simulink model "Openloop_mod"  (R2021a)
settings: Solver=VariableStepAuto  StartTime=0.0  StopTime=1  RelTol=1e-3
model workspace (MAT data in the model file):
  Vdc = 30
libraries: spsControlledVoltageSourceLib x1, spsGroundLib x1, spsPermanentMagnetSynchronousMachineLib x1, spsSawtoothGeneratorLib x1, spsThreePhaseVIMeasurementLib x1, spsUniversalBridgeLib x1, spsTriangleGeneratorLib x1, spspowerguiLib x1
settings Model: Creator=Zzx  LastModifiedBy=Zzx

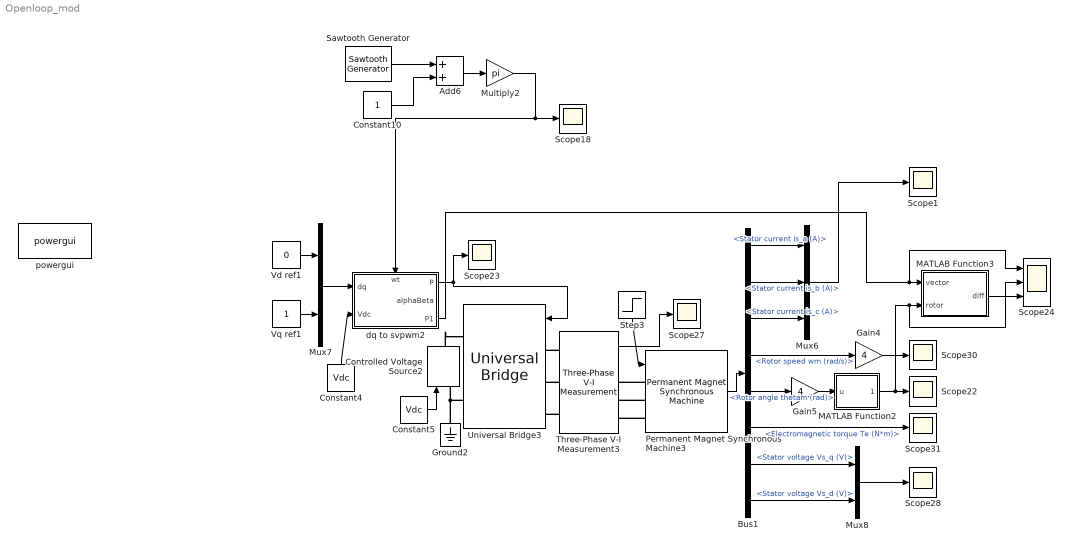
== system Openloop_mod ==
  Add6 : Sum
  Bus1 : BusSelector  OutputSignals=Stator current is_a (A),Stator current is_b (A),Stator current is_c (A),Rotor speed wm (rad/s),Rotor angle thetam (rad),Electromagnetic torque Te (N*m),Stator voltage Vs_q (V),Stator voltage Vs_d (V)
  Constant10 : Constant
  Constant4 : Constant  Value=Vdc
  Constant5 : Constant  Value=Vdc
  Controlled Voltage Source2 : spsControlledVoltageSourceLib/Controlled Voltage Source  Initialize=on  Source_Type=DC  Amplitude=0  Phase=0  Frequency=0  Measurements=Voltage
  Gain4 : Gain  Gain=4
  Gain5 : Gain  Gain=4
  Ground2 : spsGroundLib/Ground  LConnTagsString=a
  MATLAB Function2 : MATLAB Function  TreatAsAtomicUnit=on
  MATLAB Function3 : MATLAB Function  TreatAsAtomicUnit=on
  Multiply2 : Gain  Gain=pi
  Mux6 : Mux  Inputs=3
  Mux7 : Mux  Inputs=2
  Mux8 : Mux  Inputs=2
  Permanent Magnet Synchronous Machine3 : spsPermanentMagnetSynchronousMachineLib/Permanent Magnet Synchronous Machine  NbPhases=3  FluxDistribution=Sinusoidal  RotorType=Round  MechanicalLoad=Torque Tm  PresetModel=No  ShowDetailedParameters=on  MeasurementBus=off  Resistance=0.89  Inductance=8.5e-3  dqInductances=[8.5e-3,8.5e-3]  La=0.00062  MachineConstant=Voltage Constant (V_peak L-L / krpm)  Flux=0.0056925  VoltageCst=4.13  TorqueCst=0.034155  Flat=120  Mechanical=[ 0.8e-3, 0 4]  PolePairs=4  InitialConditions=[0,0, 0,0]  InitialConditions5ph=[0 0 0 0 0 0]  RefAngle=Aligned with phase A axis (original Park)  IterativeDiscreteModel=Trapezoidal non iterative  TsBlock=-1  TsPowergui=0
  Sawtooth Generator : spsSawtoothGeneratorLib/Sawtooth Generator  Freq=1  Phase=0  Ts=0
  Scope{1,18,22..23,27..28,30..31} (8 alike) : Scope
  Scope24 : Scope  NumInputPorts=3
  Step3 : Step  Time=0.5  After=0  SampleTime=0
  Three-Phase V-I Measurement3 : spsThreePhaseVIMeasurementLib/Three-Phase V-I Measurement  VoltageMeasurement=phase-to-ground  SetLabelV=off  LabelV=Vabc  Vpu=off  VpuLL=off  CurrentMeasurement=yes  SetLabelI=off  LabelI=Iabc  Ipu=off  Pbase=100e6  Vbase=500e3  OutputType=Complex  PhasorSimulation=off  PSBequivalent=0
  Universal Bridge3 : spsUniversalBridgeLib/Universal Bridge  Arms=3  SnubberResistance=1e5  SnubberCapacitance=inf  Device=IGBT / Diodes  Ron=1e-3  Lon=0  ForwardVoltages="[  0  0  ]"  ForwardVoltage=0  GTOparameters=[ 10e-6 , 20e-6 ]  IGBTparameters=[ 1e-6 , 2e-6 ]  Measurements=None  Measurements_2=None  converterType=Rectifier
  Vd ref1 : Constant  Value=0
  Vq ref1 : Constant
  dq to svpwm2 : Subsystem
      settings: PortSchema="{\"entries\":[{\"content\":{\"sides\":[{\"content\":{\"connectorIds\":[\"In1\",\"In2\"]},\"type\":\"ConnectorPlacement.EquallySpacedRectSide\",\"uuid\":\"e1c1c047-3402-4677-a9d9-6a01dbf7db4f\"},{\"content\":{\"connectorIds\":[\"Out1\",\"Out2\",\"Out3\"],\"side\":\"RIGHT\"},\"type\":\"ConnectorPlacement.EquallySpacedRectSide\",\"uuid\":\"6de788b8-e34e-4cfb-aebc-1ea17bcaea49\"},{\"content\":{\"connectorIds\":[\"In3\"],\"side\":\"TOP\"},\"type\":\"ConnectorPlacement.EquallySpacedRectSide\",\"uuid\":\"54a12e6c-3903-4ffc-a6c4-92faade7b32a\"},{\"content\":{\"connectorIds\":[],\"side\":\"BOTTOM\"},\"type\":\"ConnectorPlacement.EquallySpacedRectSide\",\"uuid\":\"2c718e0e-a6ab-4bdd-bca3-831c52d4e29e\"}]},\"type\":\"ConnectorPlacement.EquallySpacedConnector\",\"uuid\":\"b871e660-d5e9-497f-a8ea-54e97e14f77f\"}],\"packageUris\":[\"http://schema.mathworks.com/mf0/Connector/R2020b\"],\"version\":\"1.0\"}"
  powergui : spspowerguiLib/powergui  Priority=1  SimulationMode=Continuous  SampleTime=50e-6  frequency=60  Iterations=50  frequencyindice=0  Pbase=100e6  ErrMax=1e-4  UnitsV=kV  UnitsW=MW  buscounter=0  FunctionMessages=off  echomessages=off  EnableUseOfTLC=off  CurrentSourceSwitches=off  DisableSnubberDevices=off  DisableRonSwitches=off  DisableVfSwitches=off  DisplayEquations=off  AutomaticDiscreteSolvers=off  SolverType=Tustin/Backward Euler (TBE)  Interpol=off  ExternalGateDelay=off  methode=off  Ts=100  x0status=blocks  SPID=on  SwTol=0  HookPort=off  NonlinearTolerance=1e-4  nMaxIteration=100  ContinueOnMaxIteration=off  RestoreLinks=warning  ResistiveCurrentMeasurement=off  Frange=[0:2:500]  Ylog=off  Xlog=on  ShowGrid=off  save=off  variable=ZData  structure=0  ZoomFFT=off  StartTime=0.0  cycles=1  DisplayStyle=1  fundamental=60  FreqAxis=off  MaxFrequency=1000  frequencyindicesteady=1  RmsSteady=1  display=off
  wires:
  MATLAB Function3/1(diff) -> Scope24/3
  dq to svpwm2/3(P1) -> Scope24/1, MATLAB Function3/1(vector)
  Permanent Magnet Synchronous Machine3/1 -> Bus1/1
  dq to svpwm2/1(P) -> Universal Bridge3/1, Scope23/1
  MATLAB Function2/1(theta) -> Scope24/2, MATLAB Function3/2(rotor), Scope22/1
  Constant5/1 -> Controlled Voltage Source2/1
  Mux8/1 -> Scope28/1
  Bus1/1 -> Mux6/1  "<Stator current is_a (A)>"
  Vd ref1/1 -> Mux7/1
  Bus1/3 -> Mux6/3  "<Stator current is_c (A)>"
  Bus1/4 -> Gain4/1  "<Rotor speed wm (rad/s)>"
  Bus1/8 -> Mux8/2  "<Stator voltage Vs_d (V)>"
  Vq ref1/1 -> Mux7/2
  Mux7/1 -> dq to svpwm2/1(dq)
  Gain5/1 -> MATLAB Function2/1(u)
  Step3/1 -> Permanent Magnet Synchronous Machine3/1
  Bus1/5 -> Gain5/1  "<Rotor angle thetam (rad)>"
  Bus1/2 -> Mux6/2  "<Stator current is_b (A)>"
  Three-Phase V-I Measurement3/1 -> Scope27/1
  Sawtooth Generator/1 -> Add6/1
  Gain4/1 -> Scope30/1
  Add6/1 -> Multiply2/1
  Constant4/1 -> dq to svpwm2/2(Vdc)
  Multiply2/1 -> dq to svpwm2/3(wt), Scope18/1
  Constant10/1 -> Add6/2
  Bus1/6 -> Scope31/1  "<Electromagnetic torque Te (N*m)>"
  Bus1/7 -> Mux8/1  "<Stator voltage Vs_q (V)>"
  Mux6/1 -> Scope1/1
  connections:
  Universal Bridge3/RConn2 -- Controlled Voltage Source2/LConn1 -- Ground2/LConn1
  Permanent Magnet Synchronous Machine3/LConn2 -- Three-Phase V-I Measurement3/RConn2
  Three-Phase V-I Measurement3/LConn3 -- Universal Bridge3/LConn3
  Controlled Voltage Source2/RConn1 -- Universal Bridge3/RConn1
  Three-Phase V-I Measurement3/LConn2 -- Universal Bridge3/LConn2
  Permanent Magnet Synchronous Machine3/LConn3 -- Three-Phase V-I Measurement3/RConn3
  Three-Phase V-I Measurement3/LConn1 -- Universal Bridge3/LConn1
  Permanent Magnet Synchronous Machine3/LConn1 -- Three-Phase V-I Measurement3/RConn1

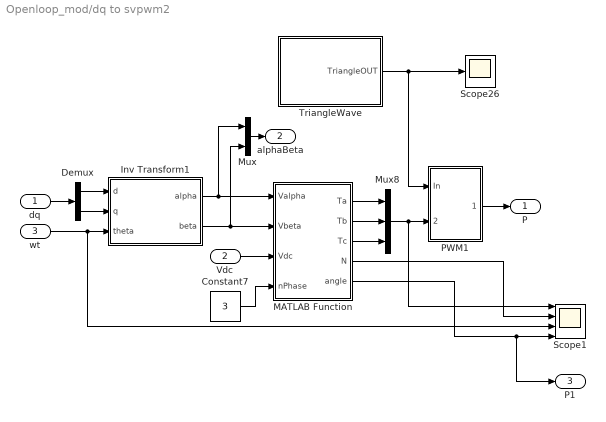
== system Openloop_mod/dq to svpwm2 ==
  dq : Inport
  Vdc : Inport  Port=2
  wt : Inport  Port=3
  Constant7 : Constant  Value=3
  Demux : Demux  Outputs=2
  Inv Transform1 : MATLAB Function  TreatAsAtomicUnit=on
  MATLAB Function : MATLAB Function  TreatAsAtomicUnit=on
  Mux : Mux  Inputs=2
  Mux8 : Mux  Inputs=3
  PWM1 : Subsystem
  Scope1 : Scope  NumInputPorts=4
  Scope26 : Scope
  TriangleWave : Subsystem
  P : Outport
  alphaBeta : Outport  Port=2
  P1 : Outport  Port=3
  wires:
  Inv Transform1/2(beta) -> MATLAB Function/2(Vbeta), Mux/2
  wt/1 -> Scope1/3, Inv Transform1/3(theta)
  dq/1 -> Demux/1
  Inv Transform1/1(alpha) -> MATLAB Function/1(Valpha), Mux/1
  MATLAB Function/1(Ta) -> Mux8/1
  MATLAB Function/3(Tc) -> Mux8/3
  MATLAB Function/2(Tb) -> Mux8/2
  Vdc/1 -> MATLAB Function/3(Vdc)
  Constant7/1 -> MATLAB Function/4(nPhase)
  PWM1/1(PWM) -> P/1
  Mux8/1 -> PWM1/2(Tcm123), Scope1/1
  Demux/1 -> Inv Transform1/1(d)
  Demux/2 -> Inv Transform1/2(q)
  Mux/1 -> alphaBeta/1
  TriangleWave/1(TriangleOUT) -> Scope26/1, PWM1/1(In)
  MATLAB Function/4(N) -> Scope1/2
  MATLAB Function/5(angle) -> P1/1, Scope1/4

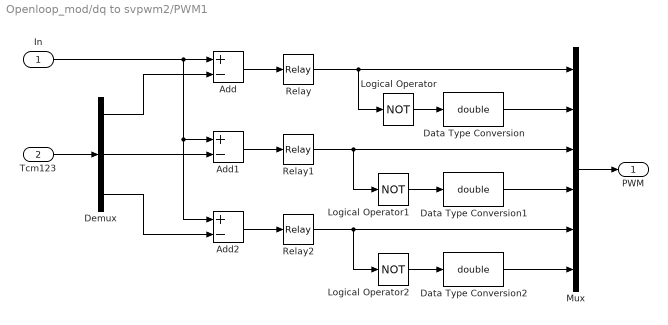
== system Openloop_mod/dq to svpwm2/PWM1 ==
  In : Inport
  Tcm123 : Inport  Port=2
  Add : Sum  Inputs=+-
  Add1 : Sum  Inputs=+-
  Add2 : Sum  Inputs=+-
  Data Type Conversion : DataTypeConversion  OutDataTypeStr=double
  Data Type Conversion1 : DataTypeConversion  OutDataTypeStr=double
  Data Type Conversion2 : DataTypeConversion  OutDataTypeStr=double
  Demux : Demux  Outputs=3
  Logical Operator : Logic  Operator=NOT  AllPortsSameDT=off  OutDataTypeStr=boolean
  Logical Operator1 : Logic  Operator=NOT  AllPortsSameDT=off  OutDataTypeStr=boolean
  Logical Operator2 : Logic  Operator=NOT  AllPortsSameDT=off  OutDataTypeStr=boolean
  Mux : Mux  Inputs=6
  Relay : Relay
  Relay1 : Relay
  Relay2 : Relay
  PWM : Outport
  wires:
  Demux/3 -> Add2/2
  Demux/2 -> Add1/2
  Demux/1 -> Add/2
  Relay2/1 -> Mux/5, Logical Operator2/1
  Relay1/1 -> Mux/3, Logical Operator1/1
  Relay/1 -> Logical Operator/1, Mux/1
  Mux/1 -> PWM/1
  Data Type Conversion/1 -> Mux/2
  Data Type Conversion1/1 -> Mux/4
  Data Type Conversion2/1 -> Mux/6
  Logical Operator2/1 -> Data Type Conversion2/1
  Logical Operator1/1 -> Data Type Conversion1/1
  Logical Operator/1 -> Data Type Conversion/1
  Add1/1 -> Relay1/1
  Add2/1 -> Relay2/1
  Add/1 -> Relay/1
  In/1 -> Add/1, Add2/1, Add1/1
  Tcm123/1 -> Demux/1

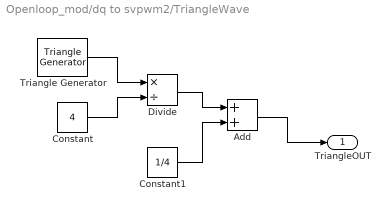
== system Openloop_mod/dq to svpwm2/TriangleWave ==
  Add : Sum
  Constant : Constant  Value=4
  Constant1 : Constant  Value=1/4
  Divide : Product  Inputs=*/
  Triangle Generator : spsTriangleGeneratorLib/Triangle Generator  Freq=f_pwm  Phase=90  Ts=0
  TriangleOUT : Outport
  wires:
  Add/1 -> TriangleOUT/1
  Constant/1 -> Divide/2
  Constant1/1 -> Add/2
  Divide/1 -> Add/1
  Triangle Generator/1 -> Divide/1

== matlab function Openloop_mod/MATLAB Function3 ==
  data: vector input; diff output; rotor input
function diff = fcn(vector,rotor)
diff = vector - rotor;
if diff < 0
    diff = vector + 2*pi - rotor;
end

== matlab function Openloop_mod/MATLAB Function2 ==
  data: u input; theta output
function theta = fcn(u)

theta = mod(u,2*pi);

== matlab function Openloop_mod/dq to svpwm2/Inv Transform1 ==
  data: d input; q input; alpha output; theta input; beta output
function [alpha,beta] = fcn(d,q,theta)

alpha = d*cos(theta)-q*sin(theta);
beta = d*sin(theta)+q*cos(theta);

== matlab function Openloop_mod/dq to svpwm2/MATLAB Function ==
  data: Valpha input; Ta output; Vbeta input; Vdc input; nPhase input; Tb output; Tc output; N output; angle output
function [Ta, Tb, Tc, N,angle ] = FindT(Valpha, Vbeta, Vdc, nPhase)
% from Valpha Vbeta calculates the 
% T0 - the idle time
% T1 - the time at Vi
% T2 - the time at V(i+1) = Vj

nPhase = floor(nPhase);
if nPhase <3
    nPhase = 3;
end

Valpha = Valpha / Vdc;
Vbeta = Vbeta/Vdc;

angle = atan2(Vbeta,Valpha);
%if Valpha<0
  %  angle = angle + pi;
%end
%angle = angle - 0.5*pi;
if angle <0
    angle = angle + 2*pi;
end

i = floor(angle/pi*nPhase);
Vi = exp(1j*pi*i/nPhase);
Vj = exp(1j*pi*(i+1)/nPhase);

Vm = (Vi+Vj)/2;
Vmabs = abs(Vm);
Vout = Valpha + 1j*Vbeta;
%Vabs = abs(Vout);

Vout_para = real(Vout * conj(Vm))/Vmabs;
if Vout_para > Vmabs
    Vout = Vout /Vout_para *Vmabs;
    Vout_para  = Vmabs;
end

T0 = 1- Vout_para / Vmabs;
Vom = Vout / Vout_para *Vmabs - Vm;
T2 = (real(Vom/(Vj-Vi))+0.5) * (1-T0);
T1 = 1-T0-T2;
N = mod(i,2*nPhase)+1;


Tall = [T0/4 T1/2+T0/4 T2/2+T0/4 T1/2+T2/2+T0/4];

switch (N)
case 1
    Ta = Tall(1);
    Tb = Tall(2);
    Tc = Tall(4);
case 2
    Ta = Tall(3);
    Tb = Tall(1);
    Tc = Tall(4);
case 3
    Ta = Tall(4);
    Tb = Tall(1);
    Tc = Tall(2);
case 4
    Ta = Tall(4);
    Tb = Tall(3);
    Tc = Tall(1);
case 5
    Ta = Tall(2);
    Tb = Tall(4);
    Tc = Tall(1);
case 6
    Ta = Tall(1);
    Tb = Tall(4);
    Tc = Tall(3);
otherwise
    Ta = 0;
    Tb = 0;
    Tc = 0;
            
end

end
